simulink model "simulation_"  (R2025b)
settings: Solver=VariableStepAuto  StartTime=0.0  StopTime=10.0  RelTol=1e-3
values from neighbouring files (symbols this model uses):
  params = struct()    [parameters.m]    (also in params.mat = )
  U = [0; 0; 0.5]    [simulation.m]
  X0 = [30; 0; 0; 0; 0; 0; 0; 3; 0; 0; 0; -30]    [simulation.m]
undefined symbols (not defined in the file or in its folder): EqM
settings Model: Creator=deepa  LastModifiedBy=deepa

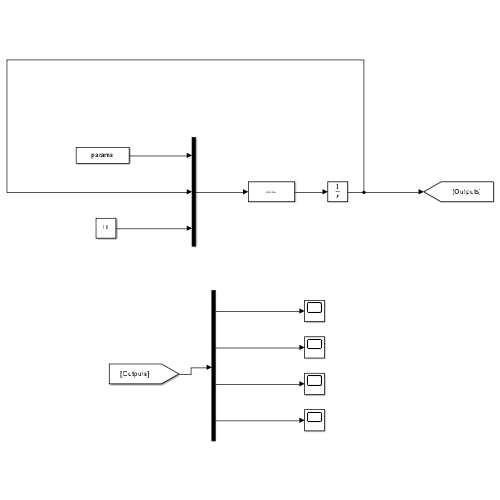
[thumbnail: Simulink's stored preview of the top-level diagram]
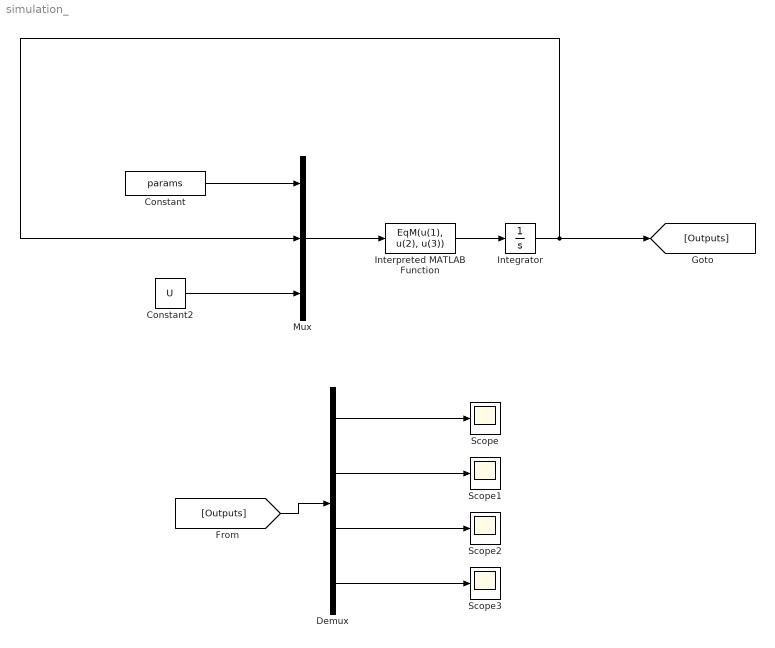
== system simulation_ ==
  Constant : Constant  Value=params
  Constant2 : Constant  Value=U
  Demux : Demux
  Integrator : Integrator  InitialCondition=X0
  Interpreted MATLAB Function : MATLABFcn  MATLABFcn=EqM(u(1), u(2), u(3))
  Mux : Mux  Inputs=3
  Scope{,1..3} (4 alike) : Scope
      Scope2 settings: DataLoggingVariableName=ScopeData2
      Scope3 settings: DataLoggingVariableName=ScopeData3
  wires:
  Constant2/1 -> Mux/3
  Integrator/1 -> [Outputs], Mux/2
  Constant/1 -> Mux/1
  Mux/1 -> Interpreted MATLAB Function/1
  Interpreted MATLAB Function/1 -> Integrator/1
  [Outputs] -> Demux/1
  Demux/1 -> Scope/1
  Demux/2 -> Scope1/1
  Demux/3 -> Scope2/1
  Demux/4 -> Scope3/1
